simulink model "CRCL"  (R2020b)
settings: Solver=FixedStepDiscrete  StartTime=0.0  StopTime=inf  FixedStep=0.01  RelTol=1e-3  EnableMultiTasking=on
values from neighbouring files (symbols this model uses):
  calibrationDelayTime_s = 2.0    [CRCL_Dictionary.sldd]
  collisionAngleThreshold_deg = 40.0    [CRCL_Dictionary.sldd]
  collisionVarianceThreshold_g2 = 8.0    [CRCL_Dictionary.sldd]
  cpMaxAbortTime_s = 30.0    [CRCL_Dictionary.sldd]
  cpMaxTipOverAngle_deg = 35.0    [CRCL_Dictionary.sldd]
  cpMinEstDistance_m = 50.0    [CRCL_Dictionary.sldd]
  cpMinEstDistanceGnssBased_m = 200.0    [CRCL_Dictionary.sldd]
  cpMinRiddenTime_s = 15.0    [CRCL_Dictionary.sldd]
  cpMinSpeedRiding_kmh = 10.0    [CRCL_Dictionary.sldd]
  cpNumCrankRevolutionThreshold = 5.0    [CRCL_Dictionary.sldd]
  cpSpeedCond2PositiveSpeedChangeTime_s = 5.0    [CRCL_Dictionary.sldd]
  cpSpeedDerivativeThreshold_kmhs = 0.005    [CRCL_Dictionary.sldd]
  cpTimeOutSpeedCond2_s = 15.0    [CRCL_Dictionary.sldd]
  groundHitEnergyThresholdStanding_g2s2 = 0.02    [CRCL_Dictionary.sldd]
  groundHitTipOverAngleThreshold_deg = 40.0    [CRCL_Dictionary.sldd]
  longAccCompForEulerEstFlag = 0.0    [CRCL_Dictionary.sldd]
  minEnergyStrongHit_g2s2 = 0.1    [CRCL_Dictionary.sldd]
  noMotionAccVarianceThresholdSD_g2 = 0.001    [CRCL_Dictionary.sldd]
  ride1minSpeedSlow_kmh = 4.0    [CRCL_Dictionary.sldd]
  ride2minSpeed_kmh = 8.0    [CRCL_Dictionary.sldd]
  rroMaxSpeed_kmh = 5.0    [CRCL_Dictionary.sldd]
  rroMinGyrX_degs = 20.0    [CRCL_Dictionary.sldd]
  rroMonotonyThreshold_degs = -1.0    [CRCL_Dictionary.sldd]
  rroRollIntegrationAngleThreshold_degs = 20.0    [CRCL_Dictionary.sldd]
  rroUniContinuityThreshold_degs = 15.0    [CRCL_Dictionary.sldd]
  scaleFactorVarianceStrongHit = 2.0    [CRCL_Dictionary.sldd]
  sdoMaxAccVarFreeFall_g2 = 0.06    [CRCL_Dictionary.sldd]
  sdoMaxTipOverAngle_deg = 20.0    [CRCL_Dictionary.sldd]
  sdoMinAccVar_g2 = 8.0    [CRCL_Dictionary.sldd]
  sdoMinGyrXYNorm_degs = 720.0    [CRCL_Dictionary.sldd]
  sdoMinGyrXYNormFreeFall_degs = 100.0    [CRCL_Dictionary.sldd]
  sdoMinOrientationChange_deg = 120.0    [CRCL_Dictionary.sldd]
  sdoScaleFactorOrientationChange = 3.0    [CRCL_Dictionary.sldd]
  stepTime_s = 0.01    [CRCL_Dictionary.sldd]
  strongHitSafetyFactor = 2.5    [CRCL_Dictionary.sldd]
  tipOverAccZFiltTreshold_g = 0.7    [CRCL_Dictionary.sldd]
  tipOverAngleThreshold_deg = 50.0    [CRCL_Dictionary.sldd]
  tipOverMinAccZFiltNoseOver_g = 0.3    [CRCL_Dictionary.sldd]
  tipOverRollPitchRelationNoseOver = 1.5    [CRCL_Dictionary.sldd]
undefined symbols (not defined in the file or in its folder): magnitude
libraries: simulink x17
(part 3 of 8)

== stateflow chart CRCL/HitDetection ==
  state GroundHitDetection [parallel]
    settings: executionOrder=1
    state Init
      en:
      %HD_LATCHTIME = 2; %sec
      HD_LATCHTIME = single(3.5); %sec
      HD_groundHitFire = int16(0);
    state waitFor10Samples
    note: pitch: 30 || roll 40
    note: ????
    state Latch
      en:
    state CheckVariance
      en:
      HD_groundHitFire = int16(0);
      du:
    (default) -> GroundHitDetection.Init
    GroundHitDetection.Init -> GroundHitDetection.waitFor10Samples
    GroundHitDetection.waitFor10Samples -> GroundHitDetection.waitFor10Samples [order 2] : % bike has to be at least one time upright before crashing !
        | [HD_curTipOverAngle_deg >= 50]
    GroundHitDetection.waitFor10Samples -> GroundHitDetection.CheckVariance [order 1] : [after(0.5,sec) && HD_secCalibDone == 1]
    GroundHitDetection.CheckVariance -> GroundHitDetection.Latch [order 1] : % riding, different angle tresholds!
        | [HD_curRideFire == 2 &&  (HD_curAccImpulseSTX^2+HD_curAccImpulseSTY^2) >= HD_groundHitEnergyThreshold * HD_groundHitScaleFactor  &&...
        | HD_curTipOverAngle_deg >= HD_groundHitAngleThreshold_deg + 5] %(abs(HD_curPitch_deg) >= 45 || abs(HD_curRoll_deg) >= 50)]
        | {
        | HD_groundHitFire = int16(1);
        | }
    GroundHitDetection.CheckVariance -> GroundHitDetection.Latch [order 2] : %riding, different angle tresholds!
        | [HD_curRideFire == 1 && ...
        | (HD_curAccImpulseSTX^2+HD_curAccImpulseSTY^2) >= HD_groundHitEnergyThresholdStanding * HD_groundHitScaleFactor  &&...
        | HD_curTipOverAngle_deg >= HD_groundHitAngleThreshold_deg]  %(abs(HD_curPitch_deg) >= 40 || abs(HD_curRoll_deg) >= 40)]
        | {
        | HD_groundHitFire = int16(1);
        | }
    GroundHitDetection.CheckVariance -> GroundHitDetection.Latch [order 3] : %not riding, different angle tresholds!
        | [HD_curRideFire == 0 && ...
        | (HD_curAccImpulseSTX^2+HD_curAccImpulseSTY^2) >= HD_groundHitEnergyThresholdStanding * HD_groundHitScaleFactor  &&...
        | HD_curTipOverAngle_deg >= HD_groundHitAngleThreshold_deg + 5] %(abs(HD_curPitch_deg) >= 40 || abs(HD_curRoll_deg) >= 40)]
        | {
        | HD_groundHitFire = int16(1);
        | }
    GroundHitDetection.Latch -> GroundHitDetection.CheckVariance : [after(HD_LATCHTIME,sec)]
        | {
        |
        | }
  state CollisionHitDetection [parallel]
    settings: executionOrder=2
    state Init
      en:
      %HD_HIT_THRESHOLD_COLLISION = single(8);	%800
      %HD_LATCHTIME = 2; %sec
      HD_LATCHTIME = single(5); %sec
      HD_collisionHitFire = int16(0);
      HD_CollisionCurVarSum = single(0);
      HD_softCollisionHitFireTmp = int16(0);
      %HD_softCollSumVarMin = 2;
      %HD_softCollSumVarMin = 2.7;
    state waitFor10Samples
    state Latch
      en:
      du:
      HD_CollisionCurVarSumTmp = HD_curVarX + HD_curVarY + HD_curVarZ;
      if HD_curRideFire >= 1
      if HD_CollisionCurVarSumTmp > HD_varScaleStrongHit * HD_collisionVarianceThreshold_g2 && ...
      (sqrt(HD_curVarY^2+HD_curVarX^2) >= 2*HD_collisionVarianceThreshold_g2) && ...
      (HD_curAccImpulseX^2+HD_curAccImpulseY^2) >= HD_CollisionEnergyThreshold*HD_strongHitSafetyfactor && ...
      (HD_curAccImpulseX^2+HD_curAccImpulseY^2) >= HD_minEnergyStrongHit_g2s2 && ...
      HD_curTipOverAngle_deg < HD_collisionAngleThreshold_deg+10
      HD_collisionHitFire = int16(3);
      end
      else
      if HD_CollisionCurVarSumTmp > HD_varScaleStrongHit * HD_collisionVarianceThreshold_g2 && ...
      (sqrt(HD_curVarY^2+HD_curVarX^2) >= 2*HD_collisionVarianceThreshold_g2) && ...
      (HD_curAccImpulseX^2+HD_curAccImpulseY^2) >= HD_CollisionEnergyThreshold*HD_strongHitSafetyfactor && ...
      (HD_curAccImpulseX^2+HD_curAccImpulseY^2) >= HD_minEnergyStrongHit_g2s2 && ...
      HD_curTipOverAngle_deg < HD_collisionAngleThreshold_deg
      HD_collisionHitFire = int16(3);
      end
      end
    state CheckVariance
      en:
      HD_CollisionCurVarSum = single(HD_curVarX + HD_curVarY + HD_curVarZ);
      du:
      HD_CollisionCurVarSum = single(HD_curVarX + HD_curVarY + HD_curVarZ);
    note: 2?
    state TimeDelayBetweenEnergyMaxAndVarianceMax
      en:
      HD_maxAccXYEnergy = HD_curAccImpulseX^2+HD_curAccImpulseY^2;
      HD_varThres = HD_varScaleStrongHit*HD_collisionVarianceThreshold_g2 * HD_CollisionEnergyThreshold*HD_strongHitSafetyfactor /  HD_maxAccXYEnergy;
      du:
      if HD_maxAccXYEnergy < (HD_curAccImpulseX^2+HD_curAccImpulseY^2)
      HD_maxAccXYEnergy = HD_curAccImpulseX^2+HD_curAccImpulseY^2;
      HD_varThres = HD_varScaleStrongHit*HD_collisionVarianceThreshold_g2 * HD_CollisionEnergyThreshold*HD_strongHitSafetyfactor /  HD_maxAccXYEnergy;
      end
      %HD_CollisionCurVarSumTmp = HD_curVarX + HD_curVarY + HD_curVarZ;
      %if HD_CollisionCurVarSumTmp > 4 * HD_collisionVarianceThreshold_g2 && ...
      %        (sqrt(HD_curVarY^2+HD_curVarX^2) >= HD_varThres) && ...
      %        abs(HD_curPitch_deg) < 40 && abs(HD_curRoll_deg) < 40
      %    HD_collisionHitFire = int16(3);
      %end
      if (sqrt(HD_curVarX^2+ HD_curVarY^2+HD_curVarZ^2) >= HD_varThres) && ...
      HD_curTipOverAngle_deg < HD_collisionAngleThreshold_deg+10
      HD_collisionHitFire = int16(3);
      end
      note: AVOID DIVISION BY ZERO!!!
      note: AVOID DIVISION BY ZERO!!!
    (default) -> CollisionHitDetection.Init
    CollisionHitDetection.Init -> CollisionHitDetection.waitFor10Samples
    CollisionHitDetection.waitFor10Samples -> CollisionHitDetection.CheckVariance : [after(0.5,sec) && HD_secCalibDone == 1]
    CollisionHitDetection.CheckVariance -> CollisionHitDetection.Latch [order 1] : %riding
        | [HD_curRideFire >= 1 && ...
        | sqrt(HD_curVarY^2+HD_curVarX^2) >= 1/16*HD_collisionVarianceThreshold_g2  && ...
        | (... (HD_curAccImpulseX^2+HD_curAccImpulseY^2) >= HD_CollisionEnergyThreshold || HD_curAccImpulseY^2 >= 2/3*HD_CollisionEnergyThreshold ||...
        | (HD_curAccImpulseX^2+HD_curAccImpulseY^2) >= HD_CollisionEnergyThreshold) && ...% 0.5*(HD_curAccImpulseX^2+HD_curAccImpulseY^2) >=  HD_curZEnergyLatched && ...abs(HD_curPitch_deg) < 45 && ...
        | HD_curTipOverAngle_deg < HD_collisionAngleThreshold_deg+5]%abs(HD_curRoll_deg) < 50 && abs(HD_curPitch_deg) < 50]
        | {
        | HD_collisionHitFire = int16(2);
        | }
    CollisionHitDetection.Latch -> CollisionHitDetection.Latch [order 3] : [(HD_curAccImpulseX^2+HD_curAccImpulseY^2) >= HD_CollisionEnergyThreshold &&...
        | HD_curTipOverFire == 0]
    CollisionHitDetection.CheckVariance -> CollisionHitDetection.Latch [order 2] : %not riding
        | [HD_curRideFire == 0 && ...
        | (sqrt(HD_curVarY^2+HD_curVarX^2) >= 1/32*HD_collisionVarianceThreshold_g2 ) && ...
        | ((HD_curAccImpulseX^2+HD_curAccImpulseY^2) >= HD_CollisionEnergyThreshold) && ...% 0.5*(HD_curAccImpulseX^2+HD_curAccImpulseY^2) >=  HD_curZEnergyLatched && ...
        | HD_curTipOverAngle_deg < HD_collisionAngleThreshold_deg] %abs(HD_curPitch_deg) < 40 && abs(HD_curRoll_deg) < 40]
        | {
        | HD_collisionHitFire = int16(2);
        | }
    CollisionHitDetection.Latch -> CollisionHitDetection.CheckVariance [order 2] : [after(HD_LATCHTIME,sec)]
        | {
        | HD_CollisionCurVarSum = single(0);
        | HD_collisionHitFire = int16(0);
        | }
    CollisionHitDetection.CheckVariance -> (junction 119) [order 5] : %passiveCrashTestsFelixBrenner
        | [HD_curVarX + HD_curVarY >= 1.5 && ...
        | HD_curTipOverFire == 0 && ...
        | HD_curTipOverAngle_deg < 35 && ...
        | (abs(HD_curAccImpulseX) >= 0.08 || ...
        | abs(HD_curAccImpulseY) >= 0.08) && ...
        | HD_curSpeed_kmh <= 3]
    CollisionHitDetection.CheckVariance -> (junction 119) [order 4] : [HD_curVarX + HD_curVarY >= 2 && ...
        | HD_curTipOverFire == 0 && ...
        | HD_curTipOverAngle_deg < 35 && ...
        | HD_curSpeed_kmh <= 3]
    CollisionHitDetection.CheckVariance -> (junction 119) [commented out] : %frontal softCollisionHit
        | [HD_curVarX + HD_curVarY >= 2.5 && ...
        | HD_curTipOverFire == 0 && ...
        | HD_curTipOverAngle_deg< 45 && ...
        | abs(HD_curAccImpulseX) >= 0.08 && ...
        | HD_curSpeed_kmh <= 3]
    (junction 119) -> CollisionHitDetection.CheckVariance : {
        | HD_softCollisionHitFireTmp = int16(1);
        | }
    CollisionHitDetection.CheckVariance -> CollisionHitDetection.CheckVariance [order 3] : [after(HD_LATCHTIME,sec)]
        | {
        | HD_softCollisionHitFireTmp = int16(0);
        | HD_collisionHitFire = int16(0);
        | }
    TimeDelayBetweenEnergyMaxAndVarianceMax -> CollisionHitDetection.Latch : [after(0.2,sec)]
        | {
        | }
    CollisionHitDetection.Latch -> TimeDelayBetweenEnergyMaxAndVarianceMax [order 1] : [(HD_curAccImpulseX^2+HD_curAccImpulseY^2) >= HD_CollisionEnergyThreshold*HD_strongHitSafetyfactor && ...
        | (HD_curAccImpulseX^2+HD_curAccImpulseY^2) >= HD_minEnergyStrongHit_g2s2 && ...
        | (HD_curAccImpulseX^2+HD_curAccImpulseY^2) > 0 && ... % For avoiding division by zero -> see red marked textboxes
        |             HD_curTipOverAngle_deg < HD_collisionAngleThreshold_deg+10]
  state HitDirectionDetection [parallel] [commented out]
    state Init [commented out]
      en:
      HD_MIN_ACC = single(2);	%2.5
      %HD_sumTIme = 0;
      HD_hitDirection = int16(0);
      HD_collisionFrontalRearLat = int16(0);
    state waitFor10Samples [commented out]
    state waitForHighAcc [commented out]
      en:
      HD_accSumX = single(0);
      HD_accSumY = single(0);
      HD_accSumZ = single(0);
      HD_accAbsSumX = single(0);
      HD_accAbsSumY = single(0);
      HD_accAbsSumZ = single(0);
      %HD_sumTime_s = single(0);
      HD_hitDirection = int16(0);
      HD_collisionFrontalRearLat = int16(0);
      HD_hitDirChangeFlag = single(0);
    state accIntegration [commented out]
      en:
    state waitForEndOfCrash1 [commented out]
    state waitForBeginningOfCrash [commented out]
    note: Execution Order!!!
    (default) -> HitDirectionDetection.Init [commented out]
    HitDirectionDetection.Init -> HitDirectionDetection.waitFor10Samples [commented out]
    HitDirectionDetection.waitFor10Samples -> HitDirectionDetection.waitForHighAcc [commented out] : [after(0.5,sec)]
    HitDirectionDetection.waitForHighAcc -> HitDirectionDetection.accIntegration [commented out] : [(abs(HD_curAccBfX) >= HD_MIN_ACC ||...
        | abs(HD_curAccBfY) >= HD_MIN_ACC || ...
        | abs(HD_curAccBfZ) >= 4*HD_MIN_ACC ) && ... % greater value for z-axis!!!
        | HD_curTipOverFire == 0]
    HitDirectionDetection.accIntegration -> HitDirectionDetection.waitForHighAcc [commented out] : [after(2,sec)]
    HitDirectionDetection.waitForBeginningOfCrash -> HitDirectionDetection.waitForHighAcc [commented out] : [after(HD_LATCHTIME+0.05,sec)]
    HitDirectionDetection.waitForEndOfCrash1 -> HitDirectionDetection.waitForHighAcc [commented out] : [HD_crashFire == 0]
    HitDirectionDetection.accIntegration -> (junction 45) [commented out] : [after(0.02,sec) && HD_collisionHitFire >= 1]
    (junction 45) -> HitDirectionDetection.accIntegration [commented out] : [HD_curAccImpulseY == 0 && HD_curAccImpulseX == 0]
    HitDirectionDetection.waitForBeginningOfCrash -> HitDirectionDetection.waitForEndOfCrash1 [commented out] : [HD_crashFire == 1]
    HitDirectionDetection.waitForBeginningOfCrash -> (junction 45) [commented out] : % update Hit Direction
        | % when strongCollisionHit appears
        | [HD_collisionHitFire >= 2 && ...
        | HD_hitDirChangeFlag == 0]
        | {
        | HD_hitDirChangeFlag = single(1);
        | }
    (junction 45) -> HitDirectionDetection.waitForBeginningOfCrash [commented out] : % bikeParkDrop or rough ground
    HitDirectionDetection.waitForBeginningOfCrash -> HitDirectionDetection.waitForBeginningOfCrash [commented out] : [HD_collisionHitFire >= 2]
    (junction 66) -> HitDirectionDetection.waitForBeginningOfCrash [commented out] : % rear Collision
        |
        | {
        | HD_hitDirection = int16(3);
        | }
    (junction 156) -> HitDirectionDetection.waitForBeginningOfCrash [commented out] : [HD_curAccImpulseY > 0]
        | {
        | HD_hitDirection = int16(2);
        | }
    (junction 66) -> HitDirectionDetection.waitForBeginningOfCrash [commented out] : % frontal Collision
        | [HD_curAccImpulseX < 0]
        | {
        | HD_hitDirection = int16(1);
        | }
    (junction 45) -> (junction 156) [commented out] : % lateral collsion
        | [abs(HD_curAccImpulseY) > abs(HD_curAccImpulseX) &&...
        | abs(HD_curAccImpulseY) > abs(HD_curAccImpulseZ)-0.1]
        | {
        | HD_collisionFrontalRearLat = int16(1);
        | }
    (junction 45) -> (junction 66) [commented out] : % frontal or rear collsion
        | {
        | HD_collisionFrontalRearLat = int16(1);
        | }
    (junction 156) -> HitDirectionDetection.waitForBeginningOfCrash [commented out] : %
        | [HD_curAccImpulseY < 0]
        | {
        | HD_hitDirection = int16(4);
        | }
  note: AVOID DIVISION BY ZERO!!!
  state CollisionSoftHitDetection [parallel]
    settings: executionOrder=3
    state Init
      en:
    state SoftCollisionTrue
      entry:
      HD_collisionHitFire = int16(1);
    state unplausibleSoftHit
      %see studentTest:
      % _ReutlingenVorne_3_MTB_40_1.-.3.2.mat
    (default) -> CollisionSoftHitDetection.Init
    unplausibleSoftHit -> CollisionSoftHitDetection.Init : [HD_softCollisionHitFireTmp == 0]
    SoftCollisionTrue -> CollisionSoftHitDetection.Init : [HD_softCollisionHitFireTmp == 0]
    CollisionSoftHitDetection.Init -> (junction 102) : [HD_softCollisionHitFireTmp == 1]
    (junction 102) -> SoftCollisionTrue [order 1] : % no change of bike attitude
        | [abs(HD_curRollDeriv) <= 20 && ...
        |  abs(HD_curPitchDeriv) <= 20]
    (junction 102) -> (junction 108) [order 2]
    (junction 108) -> SoftCollisionTrue [order 2]
    (junction 108) -> unplausibleSoftHit [order 1] : [HD_curAccYMax*HD_curRollDeriv >= 0 &&...
        | HD_curVarY >= HD_curVarX]
  state HitDirectionDetection1 [parallel]
    settings: executionOrder=4
    state Init
      en:
      HD_MIN_ACC = single(2);	%2.5
      %HD_sumTIme = 0;
      HD_hitDirection = int16(0);
      HD_collisionFrontalRearLat = int16(0);
    state waitFor10Samples
    state waitForHighAcc
      en:
      HD_accSumX = single(0);
      HD_accSumY = single(0);
      HD_accSumZ = single(0);
      HD_accAbsSumX = single(0);
      HD_accAbsSumY = single(0);
      HD_accAbsSumZ = single(0);
      %HD_sumTime_s = single(0);
      HD_hitDirection = int16(0);
      HD_collisionFrontalRearLat = int16(0);
    state accIntegration
      en:
    state waitForEndOfCrash1
    state waitForBeginningOfCrash
    state waitForMaxAmplitude
      en:
      %get max combined amplitude
      HD_maxImpulseAmplitude = sqrt(HD_curAccImpulseX^2+HD_curAccImpulseY^2);
      HD_maxImpulseXAmplitude = HD_curAccImpulseX;
      HD_maxImpulseYAmplitude = HD_curAccImpulseY;
      HD_directionTimer = 0;
      du:
      if sqrt(HD_curAccImpulseX^2+HD_curAccImpulseY^2) > HD_maxImpulseAmplitude
      HD_maxImpulseAmplitude = sqrt(HD_curAccImpulseX^2+HD_curAccImpulseY^2);
      HD_maxImpulseXAmplitude = HD_curAccImpulseX;
      HD_maxImpulseYAmplitude = HD_curAccImpulseY;
      HD_directionTimer = 0;
      else
      HD_directionTimer = HD_directionTimer + 1;
      end
      ex:
      HD_collisionFireStored = HD_collisionHitFire;
    note: Execution Order!!!
    (default) -> HitDirectionDetection1.Init
    HitDirectionDetection1.Init -> HitDirectionDetection1.waitFor10Samples
    HitDirectionDetection1.waitFor10Samples -> HitDirectionDetection1.waitForHighAcc : [after(0.5,sec)]
    HitDirectionDetection1.waitForHighAcc -> HitDirectionDetection1.accIntegration : [(abs(HD_curAccBfX) >= HD_MIN_ACC ||...
        | abs(HD_curAccBfY) >= HD_MIN_ACC || ...
        | abs(HD_curAccBfZ) >= 4*HD_MIN_ACC ) && ... % greater value for z-axis!!!
        | HD_curTipOverFire == 0]
    HitDirectionDetection1.accIntegration -> HitDirectionDetection1.waitForHighAcc [order 2] : [after(2,sec)]
    HitDirectionDetection1.waitForBeginningOfCrash -> HitDirectionDetection1.waitForHighAcc [order 1] : [after(HD_LATCHTIME+0.05,sec)]
    HitDirectionDetection1.waitForEndOfCrash1 -> HitDirectionDetection1.waitForHighAcc : [HD_crashFire == 0]
    waitForMaxAmplitude -> HitDirectionDetection1.accIntegration [order 1] : %[HD_curAccImpulseY == 0 && HD_curAccImpulseX == 0]
        | [abs(HD_curAccImpulseY) <= 0.001 && ...
        | abs(HD_curAccImpulseX) <= 0.001]
    HitDirectionDetection1.accIntegration -> waitForMaxAmplitude [order 1] : [HD_collisionHitFire >= 1]
    HitDirectionDetection1.waitForBeginningOfCrash -> HitDirectionDetection1.waitForEndOfCrash1 [order 2] : [HD_crashFire == 1]
    HitDirectionDetection1.waitForBeginningOfCrash -> HitDirectionDetection1.waitForBeginningOfCrash [order 4] : [HD_collisionHitFire >= 2]
    (default) -> HitDirectionDetection1.waitForBeginningOfCrash [commented out] : % bikeParkDrop or rough ground
    (junction 261) -> HitDirectionDetection1.waitForBeginningOfCrash [order 2] : % rear Collision
        |
        | {
        | HD_hitDirection = int16(3);
        | }
    HitDirectionDetection1.waitForBeginningOfCrash -> waitForMaxAmplitude [order 3] : % update Hit Direction
        | % when strongCollisionHit appears
        | [HD_collisionHitFire > HD_collisionFireStored]
    (junction 260) -> HitDirectionDetection1.waitForBeginningOfCrash [order 1] : [HD_maxImpulseYAmplitude > 0]
        | {
        | HD_hitDirection = int16(2);
        | }
    (junction 261) -> HitDirectionDetection1.waitForBeginningOfCrash [order 1] : % frontal Collision
        | [HD_maxImpulseXAmplitude < 0]
        | {
        | HD_hitDirection = int16(1);
        | }
    (junction 260) -> HitDirectionDetection1.waitForBeginningOfCrash [order 2] : %
        | [HD_maxImpulseYAmplitude < 0]
        | {
        | HD_hitDirection = int16(4);
        | }
    waitForMaxAmplitude -> (junction 289) [order 2] : [sqrt(HD_curAccImpulseX^2+HD_curAccImpulseY^2) <= HD_maxImpulseAmplitude*0.15 || ...
        | HD_directionTimer >= 5]
    (junction 289) -> (junction 260) [order 1] : % lateral collsion
        | [abs(HD_maxImpulseYAmplitude) > abs(HD_maxImpulseXAmplitude) &&...
        | abs(HD_maxImpulseYAmplitude) > abs(HD_curAccImpulseZ)-0.1]
        | {
        | HD_collisionFrontalRearLat = int16(1);
        | }
    (junction 289) -> (junction 261) [order 2] : % frontal or rear collsion
        | {
        | HD_collisionFrontalRearLat = int16(1);
        | }
  data: HD_curVarX input; HD_curVarY input; HD_curVarZ input; HD_groundHitFire output; HD_LATCHTIME local; HD_curTipOverFire input; HD_collisionHitFire output; HD_CollisionCurVarSum output; HD_crashFire input int16; HD_curAccBfX input; HD_curAccBfY input; HD_curAccBfZ input; HD_hitDirection output; HD_MIN_ACC local; HD_accSumX local; HD_accSumY local; HD_accSumZ local; HD_collisionFrontalRearLat output; HD_accAbsSumX local; HD_accAbsSumY local; HD_accAbsSumZ local; HD_CollisionCurVarSumTmp local; HD_curAccImpulseX input; HD_curAccImpulseY input; HD_curAccImpulseZ input; HD_curRollDeriv input; HD_curPitchDeriv input; HD_curAccYMax input; HD_softCollisionHitFireTmp output; HD_curRideFire input int16; HD_curAccImpulseSTX input; HD_curAccImpulseSTY input; HD_curSpeed_kmh input; HD_secCalibDone input; HD_CollisionEnergyThreshold input; HD_maxAccXYEnergy local; HD_varThres output; HD_groundHitEnergyThreshold input; HD_groundHitScaleFactor input; HD_curTipOverAngle_deg input; HD_maxImpulseXAmplitude local; HD_maxImpulseYAmplitude local; HD_maxImpulseAmplitude output; HD_directionTimer local; HD_collisionFireStored local; HD_groundHitEnergyThresholdStanding input; HD_groundHitAngleThreshold_deg input; HD_collisionVarianceThreshold_g2 input; HD_strongHitSafetyfactor input; HD_varScaleStrongHit input; HD_minEnergyStrongHit_g2s2 input; HD_collisionAngleThreshold_deg input

== stateflow chart CRCL/Chart ==
  state Init
    en:
    RRO_fire =int16(0);
    RRO_latchtime = single(3);
  state Init3
    en:
    RRO_fire = int16(1);
    RRO_timer1 = single(0);
    RRO_lastGyrX = RRO_curGyrX;
    du:
    if abs(RRO_curGyrX-RRO_lastGyrX) <= RRO_uniContinuityThreshold_degs && abs(RRO_curGyrX) >= RRO_minGyroX_degs && ...
    (abs(RRO_curGyrX) - abs(RRO_lastGyrX)) >= 0
    RRO_timer1 = RRO_timer1 + steptime_s;
    if RRO_timer1 >= 0.3
    RRO_longlastingMotion = int16(1);
    end
    else
    RRO_timer1 = single(0);
    end
    RRO_lastGyrX = RRO_curGyrX;
  state Init2
    en:
    RRO_lastGyrX = RRO_curGyrX;
    RRO_rollIntegrationAngle =RRO_curGyrX * steptime_s;
    du:
    RRO_lastGyrX = RRO_curGyrX;
    RRO_rollIntegrationAngle =RRO_rollIntegrationAngle + RRO_curGyrX * steptime_s;
  state Init1
    en:
    RRO_fire =int16(0);
    RRO_longlastingMotion = int16(0);
    RRO_lastGyrX = RRO_curGyrX;
    du:
    RRO_lastGyrX = RRO_curGyrX;
  (default) -> Init
  Init -> Init1
  Init3 -> Init3 [order 2] : [RRO_longlastingMotion==1]
      | {
      | RRO_longlastingMotion = int16(0);
      | }
  Init2 -> Init1 [order 1] : [abs(RRO_curGyrX-RRO_lastGyrX) > RRO_uniContinuityThreshold_degs || ...
      | abs(RRO_curGyrX) < RRO_minGyroX_degs || ...
      | (abs(RRO_curGyrX) - abs(RRO_lastGyrX)) < RRO_monotonyThreshold_degs]
  Init2 -> Init3 [order 2] : [after(0.3,sec) && ...
      | abs(RRO_rollIntegrationAngle) >= ...
      | RRO_rollIntegrationAngleThreshold_degs]
  Init1 -> Init2 : [abs(RRO_curGyrX-RRO_lastGyrX) <= RRO_uniContinuityThreshold_degs && ...
      | abs(RRO_curGyrX) >= RRO_minGyroX_degs && ...
      |  (abs(RRO_curGyrX) - abs(RRO_lastGyrX)) >= 0 && RRO_curSpeed_kmh <= RRO_maxSpeed_kmh]
  Init3 -> Init1 [order 1] : [after(RRO_latchtime,sec)]
  data: RRO_curGyrX input; RRO_fire output; RRO_latchtime local; RRO_lastGyrX local; steptime_s input; RRO_timer1 local; RRO_longlastingMotion local; RRO_curSpeed_kmh input; RRO_rollIntegrationAngle output; RRO_minGyroX_degs input; RRO_uniContinuityThreshold_degs input; RRO_maxSpeed_kmh input; RRO_monotonyThreshold_degs input; RRO_rollIntegrationAngleThreshold_degs input

== stateflow chart CRCL/SmartphoneDropOut_SDO ==
  state SmartphoneDropOut [parallel]
    settings: executionOrder=1
    state init
      en:
      SDO_fire = uint8(0);
      SDO_deltaRoll_deg = single(0);
      SDO_deltaPitch_deg = single(0);
      SDO_rollMin = single(0);
      SDO_rollMax = single(0);
      SDO_pitchMin = single(0);
      SDO_pitchMax = single(0);
      SDO_deltaRollExtrema_deg = single(0);
      SDO_deltaPitchExtrema_deg = single(0);
      SDO_deltaRollPitch_deg = single(0);
    state idle
      en:
      SDO_fire = uint8(0);
    state possibleCollision
      entry:
      SDO_gyrXYnorm = sqrt(SDO_curGyroBfX^2 + SDO_curGyroBfY^2);
      during:
      SDO_gyrXYnorm = sqrt(SDO_curGyroBfX^2 + SDO_curGyroBfY^2);
    state waitState
    state gyroIntegration
      entry:
      SDO_gyrXYnorm = sqrt(SDO_curGyroBfX^2 + SDO_curGyroBfY^2);
      SDO_deltaRoll_deg = SDO_curGyroBfX * SDO_timestep;
      SDO_deltaPitch_deg = SDO_curGyroBfY * SDO_timestep;
      SDO_rollMin = single(0);
      SDO_rollMax = single(0);
      SDO_pitchMin = single(0);
      SDO_pitchMax =single(0);
      SDO_minAccVarSum = SDO_curAccVarXYZ;
      during:
      SDO_gyrXYnorm = sqrt(SDO_curGyroBfX^2 + SDO_curGyroBfY^2);
      SDO_deltaRoll_deg = SDO_deltaRoll_deg + SDO_curGyroBfX * SDO_timestep;
      SDO_deltaPitch_deg = SDO_deltaPitch_deg + SDO_curGyroBfY * SDO_timestep;
      %update extrema
      if SDO_deltaRoll_deg > SDO_rollMax
      SDO_rollMax = SDO_deltaRoll_deg;
      elseif SDO_deltaRoll_deg < SDO_rollMin
      SDO_rollMin = SDO_deltaRoll_deg;
      end
      if SDO_deltaPitch_deg > SDO_pitchMax
      SDO_pitchMax = SDO_deltaPitch_deg;
      elseif SDO_deltaPitch_deg < SDO_pitchMin
      SDO_pitchMin = SDO_deltaPitch_deg;
      end
      if SDO_curAccVarXYZ < SDO_minAccVarSum && SDO_gyrXYnorm >= SDO_minGyrXYNormFreeFall_degs
      SDO_minAccVarSum = SDO_curAccVarXYZ;
      end
      %take delta between min and max angle
      SDO_deltaRollExtrema_deg = SDO_rollMax - SDO_rollMin;
      SDO_deltaPitchExtrema_deg = SDO_pitchMax - SDO_pitchMin;
      SDO_deltaRollPitch_deg = sqrt(SDO_deltaRollExtrema_deg^2+SDO_deltaPitchExtrema_deg^2);
    state wait4StandDetection
      entry:
      SDO_fire = uint8(1);
      during:
      if SDO_StandDetectionFire >= 1
      SDO_fire = uint8(2);
      end
    note: AVOID DIVISION BY ZERO!!!
        | -> USE max-function
    (default) -> init
    init -> idle
    idle -> possibleCollision : %
        | [SDO_curAccVarXYZ >=SDO_minAccVar_g2]
    possibleCollision -> idle [order 1] : [after(5,sec)]
    waitState -> idle : [after(3,sec) && SDO_curSpeed_kmh < SDO_ride1minSpeed_kmh]
    wait4StandDetection -> idle [order 2] : [after(10,sec)]
    gyroIntegration -> idle [order 1] : [after(1,sec)]
    possibleCollision -> gyroIntegration [order 2] : [ SDO_gyrXYnorm >= SDO_minGyrXYNorm_degs]
    wait4StandDetection -> waitState [order 1] : [SDO_fire >= 2]
    gyroIntegration -> wait4StandDetection [order 2] : [(SDO_deltaRollPitch_deg >= SDO_minOrientationChange_deg && ...
        | SDO_minAccVarSum <= 0.03*SDO_deltaRollPitch_deg/max(SDO_minOrientationChange_deg,1) && ...
        | SDO_minAccVarSum <= SDO_maxAccVarFreeFall_g2) ||...
        | SDO_deltaRollPitch_deg >= SDO_scaleFactorOrientationChange * ...
        | SDO_minOrientationChange_deg]
  state BikeUprightDetection [parallel]
    settings: executionOrder=2
    state Idle
      en:
      SDO_bikeUpright = uint16(0);
    state BikeUpright
    state BikeUprightValidated
      en:
      SDO_bikeUpright = uint16(1);
    (default) -> Idle
    Idle -> BikeUpright : [SDO_tipOverAngle_deg < SDO_maxTipOverAngle_deg]
    BikeUpright -> BikeUprightValidated [order 2] : [after(5,sec)]
    BikeUpright -> Idle [order 1] : [SDO_tipOverAngle_deg >= SDO_maxTipOverAngle_deg]
    BikeUprightValidated -> Idle : [SDO_tipOverAngle_deg >= 45]
  data: SDO_timestep input; SDO_curGyroBfX input; SDO_curGyroBfY input; SDO_deltaRoll_deg output; SDO_deltaPitch_deg output; SDO_fire output; SDO_gyrXYnorm output; SDO_StandDetectionFire input; SDO_rollMin local; SDO_rollMax local; SDO_pitchMin local; SDO_pitchMax local; SDO_deltaRollExtrema_deg output; SDO_deltaPitchExtrema_deg output; SDO_deltaRollPitch_deg output; SDO_curAccVarXYZ input; SDO_minAccVarSum output; SDO_curSpeed_kmh input; SDO_bikeUpright output; SDO_tipOverAngle_deg input; SDO_maxTipOverAngle_deg input; SDO_minAccVar_g2 input; SDO_minGyrXYNorm_degs input; SDO_minOrientationChange_deg input; SDO_scaleFactorOrientationChange input; SDO_maxAccVarFreeFall_g2 input; SDO_minGyrXYNormFreeFall_degs input; SDO_ride1minSpeed_kmh input

== matlab function CRCL/MATLAB Function ==
  data: pitch_deg output; timeStep_s input; accBfX_g input; roll_deg output; accBfY_g input; accBfZ_g input; gyrX_degs input; gyrY_degs input; gyrZ_degs input; innovationPitch output; innovationRoll output; pitchGyroPredict output; rollGyroPredict output; pitchAcc output; rollAcc output; gyrBiasX output; gyrBiasY output; reinitializeFlag input; SD_fire input; HD_GroundHit input; HD_CollisionHit input; TO_fire input; varSum input; accBfFiltX_g input; accBfFiltY_g input; accBfFiltZ_g input; u1 output; secondCalibrationIsDone input; u2 output
function [pitch_deg, roll_deg, innovationPitch, innovationRoll, ...
    pitchGyroPredict, rollGyroPredict, pitchAcc, rollAcc, ...
    gyrBiasX, gyrBiasY, u1, u2] ...
    = kalman1(timeStep_s, accBfX_g, accBfY_g, accBfZ_g, ...
    gyrX_degs, gyrY_degs, gyrZ_degs, reinitializeFlag, ...
    SD_fire, HD_GroundHit, HD_CollisionHit, TO_fire, varSum, ...
    accBfFiltX_g, accBfFiltY_g, accBfFiltZ_g, secondCalibrationIsDone)

%accBf_g = [accBfX_g; accBfY_g; accBfZ_g];
accBf_g = [accBfFiltX_g; accBfFiltY_g; accBfFiltZ_g];
accBf_g = accBf_g/norm(accBf_g);

%check Data: if Accelerometer is all zero, Kalman Filter returns NaN
if abs(accBf_g(1)) < 0.0001 && ...         %~any(accBf_g) 
        abs(accBf_g(2)) < 0.0001 && ...
        abs(accBf_g(3)) < 0.0001 
    accBf_g = single([0.05; 0.05; 1]);
end

dt = timeStep_s;


persistent x P A B H R Q I betaGyroBias gyrBiasMeasuredX gyrBiasMeasuredY ...
    lastAccPitch lastAccRoll

%% declaration only during first run!

if isempty(x)
    noise_accel = single(1e-1);  %1e-1
    noise_gyro = single(8e-7);   %5e-7
    x = single([0; 0]);      % Initial State (pitch and roll angle)
    P = single([1000, 0;...
        0, 1000]);       % Initial Uncertainty
    A = single([1, 0;...
        0, 1]);        % Transition Matrix
    B = single([dt, 0; ...
        0, dt]);         %control matrix -> gyro input evaluation
    H = single([1, 0; ...
        0, 1]);       % Measurement function
    R = single([noise_accel, 0;...
        0, noise_accel]);             % measurement noise covariance
    Q = single([noise_gyro, 0;...
        0, noise_gyro]); % Process Noise Covariance
    I = single(eye(2));             % Identity matrix
    gyrBiasMeasuredX = single(0);
    gyrBiasMeasuredY = single(0);
    betaGyroBias = single(1e-7);  
    lastAccPitch = single(0);
    lastAccRoll = single(0);
end

gyrBf_degs = [gyrX_degs-gyrBiasMeasuredX; gyrY_degs-gyrBiasMeasuredY; gyrZ_degs];

if reinitializeFlag == 1
    noise_accel = single(5e-3);
    R_intern = single([noise_accel, 0;...
        0, noise_accel]);   
elseif SD_fire && (HD_GroundHit == 1 || HD_CollisionHit >= 2 || TO_fire >= 2)
    noise_accel = single(5e-4);
    R_intern = single([noise_accel, 0;...
        0, noise_accel]);  
elseif varSum < 0.0002
    noise_accel = single(5e-3);
    R_intern = single([noise_accel, 0;...
        0, noise_accel]);  
else
    R_intern = R;
end

if varSum > 0.0001 || sum(abs(x)) > 20
    betaGyroBiasIntern = betaGyroBias;
else
    betaGyroBiasIntern = single(5e-6);
end

Q_intern = Q;
% if  badEulerEstimationCounter >=  5000
%     noise_gyro = single(1e-4);   %5e-7
%      Q_intern = single([noise_gyro, 0;...
%         0, noise_gyro]); % Process Noise Covariance
%     noise_accel = single(5e-5);
%     R_intern = single([noise_accel, 0;...
%         0, noise_accel]);   
%     accBf_g = [accBfFiltX_g; accBfFiltY_g; accBfFiltZ_g];
% else 
%     Q_intern = Q;
% end
    
% gyro input data    
% u = [gyrY_degs-gyrBiasMeasuredY;gyrX_degs-gyrBiasMeasuredX];
% u = [(gyrY_degs-gyrBiasMeasuredY)*cosd(x(2))-gyrZ_degs*sind(x(2)); ...
%    gyrX_degs-gyrBiasMeasuredX];
% u = [(gyrY_degs-gyrBiasMeasuredY)*cosd(x(2))-gyrZ_degs*sind(x(2)); ...
%     (gyrX_degs-gyrBiasMeasuredX)*cosd(x(1))-gyrZ_degs*sind(x(1))];



%rotate Data into navigation frame see: https://de.wikipedia.org/wiki/Eulersche_Winkel
gyrNf_degs = [cosd(x(1)) 0 sind(x(1)); ...
    0 1 0; ...
    -sind(x(1)) 0 cosd(x(1))] * ...
    [1 0 0; ...
    0 cosd(x(2)) -sind(x(2));
    0 sind(x(2)) cosd(x(2))] * gyrBf_degs;

u=[gyrNf_degs(2); gyrNf_degs(1)];
u1 = u(1);
u2 = u(2);

% Prediction    
x_predict = A * x + B * u;                  % Prädizierter Zustand aus Bisherigem und System
P = A * P * A' + Q_intern;             % Prädizieren der Kovarianz


% quatAcc = [0 accBf_g'];
% quatAcc = quatAcc./norm(quatAcc);
% euler = quatern2euler(quatAcc)*180/pi;
% rollAcc = euler(1);
% pitchAcc = euler(2);

%calculate acc based roll and pitch angles

denominatorRollAcc = sqrt(accBf_g(3)*accBf_g(3)+accBf_g(1)*accBf_g(1));
%AVOID DIVISION BY ZERO!
if denominatorRollAcc <= 0.0001    
    denominatorRollAcc = single(0.001);
end
rollAcc = atand(accBf_g(2)/denominatorRollAcc);
if accBf_g(3) < - 0.3 && abs(accBf_g(1)) < 0.6 && accBf_g(2) > 0 && abs(lastAccPitch) < 100
    rollAcc = -rollAcc+180;  
elseif accBf_g(3) < - 0.3 && abs(accBf_g(1)) < 0.6 && accBf_g(2) < 0 && abs(lastAccPitch) < 100
    rollAcc = -rollAcc-180; 
elseif accBf_g(1) < -0.1 && abs(accBf_g(1)) > abs(accBf_g(3))
    %rollAcc = -1*rollAcc;  
end


denominatorPitchAcc = sqrt(accBf_g(3)*accBf_g(3)+accBf_g(2)*accBf_g(2));
%AVOID DIVISION BY ZERO!
if denominatorPitchAcc < 0.0001
   denominatorPitchAcc = single(0.0001);
end
pitchAcc = -1*atand(accBf_g(1)/denominatorPitchAcc);
if accBf_g(3) < -0.3 && abs(accBf_g(2)) < 0.6 && accBf_g(1) > 0 && abs(lastAccRoll) < 100
    pitchAcc = -pitchAcc-180;
elseif accBf_g(3) < -0.3 && abs(accBf_g(2)) < 0.6 && accBf_g(1) < 0 && abs(lastAccRoll) < 100
    pitchAcc = -pitchAcc+180;
elseif accBf_g(3) < 0 && accBf_g(1) < 0
    %pitchAcc = -1*pitchAcc;
end


% Correction

Z = [pitchAcc; rollAcc];
y = Z - (H * x_predict);              % Innovation aus Messwertdifferenz
%y = Z - x_predict;     
S = (H * P * H' + R_intern);           % Innovationskovarianz
K = P * H' * inv(S);          % Filter-Matrix (Kalman-Gain)

x = x_predict + (K * y);              % aktualisieren des Systemzustands
P = (I - (K * H)) * P;          % aktualisieren der Kovarianz


%Bias Estimation
if secondCalibrationIsDone == 1 && sqrt(x_predict(1)^2+x_predict(2)^2) <= 25 && ...
        sqrt((x(1) - pitchAcc)^2 + (x(2) - rollAcc)^2) <= 30
    gyrBiasMeasuredY = (1-betaGyroBiasIntern) * gyrBiasMeasuredY + betaGyroBiasIntern*(x(1) - pitchAcc)/dt;
    gyrBiasMeasuredX = (1-betaGyroBiasIntern)  * gyrBiasMeasuredX + betaGyroBiasIntern*(x(2) - rollAcc)/dt;
    %max gyro bias of bmi160 is declared as 3°/s -> saturate bias
    %estimation, in case of misfunction
    gyrBiasMeasuredX = saturateKalman(gyrBiasMeasuredX, 4);  
    gyrBiasMeasuredY = saturateKalman(gyrBiasMeasuredY, 4);
end

pitchGyroPredict = x_predict(1);
rollGyroPredict = x_predict(2);

innovationPitch = y(1);
innovationRoll = y(2);

%unwrap pitchAngle
if x(1) > 180 
    x(1) = x(1)-360;    
elseif x(1) < -180
    x(1) = x(1)+360;
elseif (x(1) > 165 && pitchAcc < -165) || (x(1) < -165 && pitchAcc > 165)
    x(1) = -x(1); 
end

%unwrap rollAngle
if x(2) > 180 
    x(2) = x(2)-360;   
elseif x(2) < -180 
    x(2) = x(2)+360;
elseif (x(2) > 165 && rollAcc < -165) || (x(2) < -165 && rollAcc > 165)
    x(2) = -x(2); 
end

pitch_deg = x(1);
roll_deg = x(2);

gyrBiasX = gyrBiasMeasuredX;
gyrBiasY = gyrBiasMeasuredY;

debugOut = single(0);

lastAccRoll = rollAcc;
lastAccPitch = pitchAcc;

end


function euler = quatern2euler(q)
%QUATERN2EULER Converts a quaternion orientation to ZYX Euler angles
%
%   q = quatern2euler(q)
%
%   Converts a quaternion orientation to ZYX Euler angles where phi is a
%   rotation around X, theta around Y and psi around Z.
%
%   For more information see:
%   http://www.x-io.co.uk/node/8#quaternions
%
%	Date          Author          Notes
%	27/09/2011    SOH Madgwick    Initial release
% R = zeros(3,3,1);
%     R(1,1,:) = 2.*q(:,1).^2-1+2.*q(:,2).^2;
%     R(2,1,:) = 2.*(q(:,2).*q(:,3)-q(:,1).*q(:,4));
%     R(3,1,:) = 2.*(q(:,2).*q(:,4)+q(:,1).*q(:,3));
%     R(3,2,:) = 2.*(q(:,3).*q(:,4)-q(:,1).*q(:,2));
%     R(3,3,:) = 2.*q(:,1).^2-1+2.*q(:,4).^2;
% 
%     phi = atan2(R(3,2,:), R(3,3,:) );
%     theta = -atan(R(3,1,:) ./ sqrt(1-R(3,1,:).^2) );
%     psi = atan2(R(2,1,:), R(1,1,:) );
% 
%     euler = [phi(1,:)' theta(1,:)' psi(1,:)'];
    
    R = zeros(3,3);
    R(1,1) = 2.*q(1).^2-1+2.*q(2).^2;
    R(2,1) = 2.*(q(2).*q(3)-q(1).*q(4));
    R(3,1) = 2.*(q(2).*q(4)+q(1).*q(3));
    R(3,2) = 2.*(q(3).*q(4)-q(1).*q(2));
    R(3,3) = 2.*q(1).^2-1+2.*q(4).^2;

    phi = atan2(R(3,2), R(3,3));
    theta = -atan(R(3,1) ./ sqrt(1-R(3,1).^2) );
    psi = atan2(R(2,1), R(1,1) );

    euler = [phi theta psi];
end

function output = saturateKalman(input, limit)
%output = single(0);
 if input > limit
     output = single(limit);
 elseif input < -1*limit
     output = single(-1*limit);
 else
     output = single(input);
 end

end
